simulink model "Aero_Dynamics"  (Simulink 8.3)
settings: Solver=ode45  StartTime=0.0  StopTime=10.0  RelTol=1e-3
values from neighbouring files (symbols this model uses):
  AD = [0.05526	0.05526	0.05568	0.05804	0.06460	0.08210 ... (first row only)    [AirCraftData.m]
  Alpha0 = [0.143	0.143	0.122	-0.267	-0.627	0.120 ... (first row only)    [AirCraftData.m]
  CA = 3.451    [AirCraftData.m]    (also in AircraftTrim.m)
  CDmin = [0.03799	0.03799	0.03799	0.03799	0.03904	0.04277 ... (first row only)    [AirCraftData.m]
  CLAlpha = [0.1012	0.1021	0.1033	0.1051	0.1079	0.0976 ... (first row only)    [AirCraftData.m]
  Clbt0 = [-0.00147	-0.00148	-0.00149	-0.00153	-0.00158	-0.00171 ... (first row only)    [AirCraftData.m]
  Clbtaf = [0	0	0	0	0	0;0	 0	0	0	0	0]    [AirCraftData.m]
  ClDelA = [-0.003110	-0.003065	-0.003040	-0.003036	-0.003052	-0.003088 ... (first row only)    [AirCraftData.m]
  CLDelE = [0.00653	0.00668	0.00690	0.00724	0.00772	0.00846 ... (first row only)    [AirCraftData.m]
  ClDelR = [0.000584	0.000605	0.000638	0.000686	0.000760	0.000877 ... (first row only)    [AirCraftData.m]
  CLDM = [0.244	0.244	0.244	0.244	0.244	0.244 ... (first row only)    [AirCraftData.m]
  Clp0 = [-0.5510 	-0.5610 	-0.5767 	-0.6005 	-0.6224 	-0.6763 ... (first row only)    [AirCraftData.m]
  ClpAf = [0,0,0,0,0,0;0,0,0,0,0,0]    [AirCraftData.m]
  Clr0 = [0.1308 	0.1339 	0.1383 	0.1474 	0.1601 	0.1738 ... (first row only)    [AirCraftData.m]
  ClrAf = [0,0,0,0,0,0;0,0,0,0,0,0]    [AirCraftData.m]
  Cm0 = [0.2014	0.2017	0.2034	0.2083	0.2207	0.2475 ... (first row only)    [AirCraftData.m]
  CmAfdot = [-11.5890 	-12.0169 	-12.7558 	-13.8010 	-15.2088 	-16.2278 ... (first row only)    [AirCraftData.m]
  CmCl = [-0.3454	-0.3441	-0.3427	-0.3412	-0.3396	-0.3379 ... (first row only)    [AirCraftData.m]
  CmDelE = [-0.03554	-0.03651	-0.03802	-0.04028	-0.04365	-0.04798 ... (first row only)    [AirCraftData.m]
  Cmq0 = [-42.0260 	-42.2665 	-42.9499 	-44.8315 	-45.5877 	-46.0842 ... (first row only)    [AirCraftData.m]
  CN1A0 = [0.0740	0.0662	0.0605	0.0552	0.0554 ... (first row only)    [AirCraftData.m]
  Cnbt0 = [0.00180	0.00183	0.00187	0.00192	0.00200	0.00207 ... (first row only)    [AirCraftData.m]
  Cnbtaf = [-0.000030 	-0.000031 	-0.000031 	-0.000032 	-0.000033 	-0.000035 ... (first row only)    [AirCraftData.m]
  CnDelA0 = [-0.000180	-0.000178	-0.000176	-0.000176	-0.000177	-0.000179 ... (first row only)    [AirCraftData.m]
  CnDelAAf = [0	 0	0	0	0	0;0	 0	0	0	0	0]    [AirCraftData.m]
  CnDelR = [-0.002214	-0.002274	-0.002367	-0.002505	-0.002712	-0.003039 ... (first row only)    [AirCraftData.m]
  Cnp0 = [0.0521 	0.0532 	0.0571 	0.0601 	0.0636 	0.0664 ... (first row only)    [AirCraftData.m]
  CnpAf = [0,0,0,0,0,0;0,0,0,0,0,0]    [AirCraftData.m]
  Cnr = [-0.1810 	-0.1832 	-0.1855 	-0.1892 	-0.1933 	-0.1973 ... (first row only)    [AirCraftData.m]
  Cxh_Slip = [0.0000, 0.0045, 0.0089, 0.0132, 0.0174 ... (first row only)    [AirCraftData.m]
  Cybeta0 = [-0.01783	-0.01790	-0.01804	-0.01824	-0.01851	-0.01884 ... (first row only)    [AirCraftData.m]
  Cybtaf = [0 0 0 0 0 0;0 0 0 0 0 0]    [AirCraftData.m]
  CyDelA = [0.000287	0.000295	0.000307	0.000325	0.000351	0.000394 ... (first row only)    [AirCraftData.m]
  CyDelR = [0.004946	0.005035	0.005316	0.005791	0.006458	0.007318 ... (first row only)    [AirCraftData.m]
  Cyh_Slip = [0.0000, -0.0248, -0.0519, -0.0813, -0.1130 ... (first row only)    [AirCraftData.m]
  ETA_data = [0.729 0.727 0.72 0.71 0.877 0.858 0.855 0.853 0.857 0.862 0.87 0.796 ... (330 elements, 11x5x6)]    [ETA_data.mat]
  eul_0 = [0/57.3 0/57.3 0/57.3]    [AircraftTrim.m]
  flap = 0    [AircraftTrim.m]
  inertia = [  Ix      Iy     Iz  Ixz]    [AircraftTrim.m]
  mass = 54000    [Start.m]    (also in drl_simplified_dynamics.m)
  Vab_0 = [Vt 0 0]    [AircraftTrim.m]
  Wxyz_0 = [0 0 0]    [AircraftTrim.m]
  X = 1.06    [AircraftTrim.m]
  xme_0 = [0 0 -alt]    [AircraftTrim.m]
  Y = 1.177    [AircraftTrim.m]
undefined symbols (not defined in the file or in its folder): slselsubs, thrust_data
libraries: aerolibatmos2 x1, aerolibobsolete x1, aerolibutil x1
(part 1 of 2)
settings Model: Creator=Administrator  LastModifiedBy=HP  BufferReuse=off
settings OptimizationCC: InlineParams=on  BufferReuse=off  ExpressionDepthLimit=2147483647  InitFltsAndDblsToZero=on
settings DebuggingCC: AlgebraicLoopMsg=none  SaveWithParameterizedLinksMsg=none  SignalResolutionControl=TryResolveAllWithWarning  SolverPrmCheckMsg=none  MultiTaskDSMMsg=warning  MultiTaskCondExecSysMsg=none  FcnCallInpInsideContextMsg=UseLocalSettings  UnconnectedInputMsg=none  UnconnectedOutputMsg=none  UnconnectedLineMsg=none  StrictBusMsg=Warning
settings RTWCC: IncludeERTFirstTime=on
settings GRTTargetCC: TargetFcnLib=ansi_tfl_tmw.mat

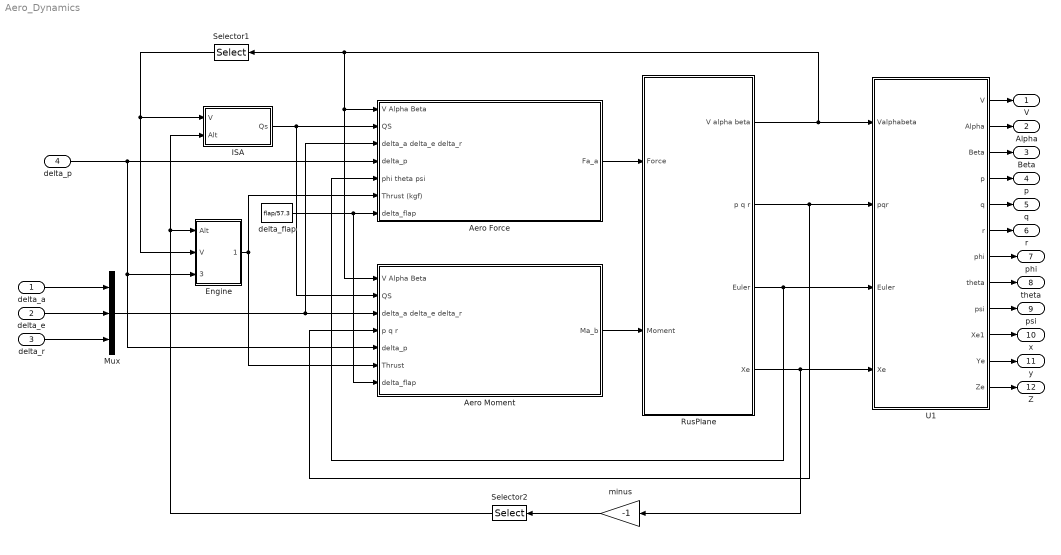
== system Aero_Dynamics ==
  delta_a : Inport
  delta_e : Inport  Port=2
  delta_r : Inport  Port=3
  delta_p : Inport  Port=4
  Aero Force : Subsystem
  Aero Moment : Subsystem
  Engine : Subsystem
  ISA : Subsystem
  Mux : Mux  Inputs=3
  RusPlane : Subsystem  mask{Xme_0=xme_0, Vab_0=Vab_0, eul_0=eul_0, Wxyz_0=Wxyz_0, inertia=inertia, mass=mass}
      mask prompts: Xme_0 "Initial position in inertial axes[Xe,Ye,Ze]"; Vab_0 "Initial velocity in body axes"; eul_0 "Initial Euler orientation"; Wxyz_0 "Initial body rotation rates"
  Selector1 : Selector  InputPortWidth=3  Indices=[1]  OutputSizes=[(-2)]
  Selector2 : Selector  InputPortWidth=3  Indices=[3]  OutputSizes=[(-2)]
  U1 : Subsystem
  delta_flap : Constant  Value=flap/57.3
  minus : Gain  Gain=-1
  V : Outport
  Alpha : Outport  Port=2
  Beta : Outport  Port=3
  p : Outport  Port=4
  q : Outport  Port=5
  r : Outport  Port=6
  phi : Outport  Port=7
  theta : Outport  Port=8
  psi : Outport  Port=9
  x : Outport  Port=10
  y : Outport  Port=11
  Z : Outport  Port=12
  wires:
  Aero Force/1(Fa_a) -> RusPlane/1(Force)
  Aero Moment/1(Ma_b) -> RusPlane/2(Moment)
  minus/1 -> Selector2/1
  RusPlane/1(V alpha beta) -> Aero Moment/1(V Alpha Beta), Aero Force/1(V Alpha Beta), Selector1/1, U1/1(Valphabeta)
  RusPlane/2(p q r) -> Aero Moment/4(p q r), U1/2(pqr)
  RusPlane/3(Euler) -> Aero Force/5(phi theta psi), U1/3(Euler)
  RusPlane/4(Xe) -> minus/1, U1/4(Xe)
  Selector1/1 -> ISA/1(V), Engine/2(V)
  ISA/1(Qs) -> Aero Force/2(QS), Aero Moment/2(QS)
  Engine/1(Thrust) -> Aero Force/6(Thrust (kgf)), Aero Moment/6(Thrust)
  Selector2/1 -> ISA/2(Alt), Engine/1(Alt)
  delta_a/1 -> Mux/1
  delta_e/1 -> Mux/2
  delta_r/1 -> Mux/3
  Mux/1 -> Aero Moment/3(delta_a delta_e delta_r), Aero Force/3(delta_a delta_e delta_r)
  delta_p/1 -> Aero Force/4(delta_p), Aero Moment/5(delta_p), Engine/3(delta_p)
  delta_flap/1 -> Aero Force/7(delta_flap), Aero Moment/7(delta_flap)
  U1/1(V) -> V/1
  U1/2(Alpha) -> Alpha/1
  U1/3(Beta) -> Beta/1
  U1/4(p) -> p/1
  U1/5(q) -> q/1
  U1/6(r) -> r/1
  U1/7(phi) -> phi/1
  U1/8(theta) -> theta/1
  U1/9(psi) -> psi/1
  U1/10(Xe1) -> x/1
  U1/11(Ye) -> y/1
  U1/12(Ze) -> Z/1

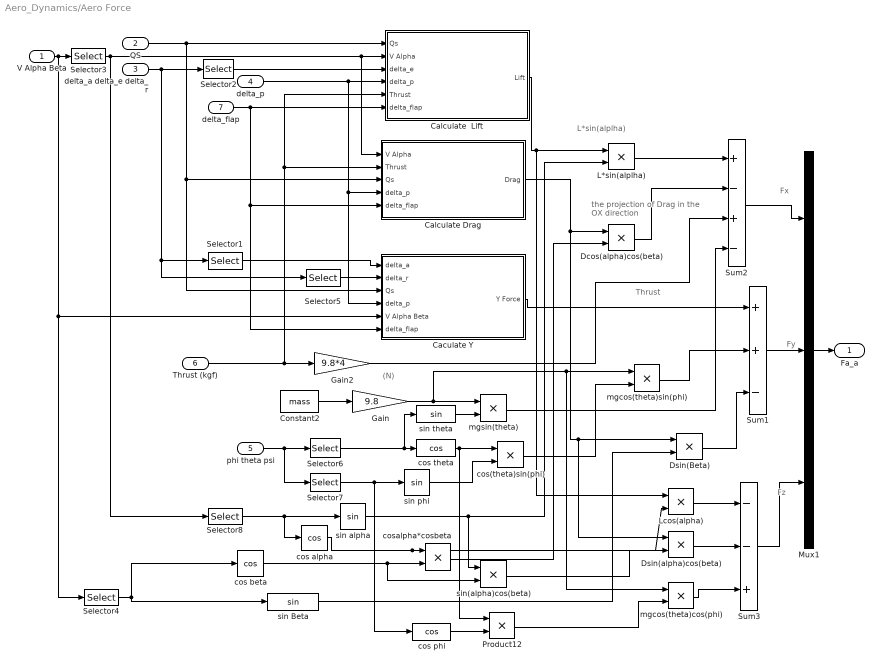
== system Aero_Dynamics/Aero Force ==
  note: Fx
  note: L*sin(alplha)
  note: the projection of Drag
      | in the OX direction
  note: Fy
  note: Fz
  note: Thrust
  note: (N)
  V Alpha Beta : Inport
  QS : Inport  Port=2
  delta_a delta_e delta_r : Inport  Port=3
  delta_p : Inport  Port=4
  phi theta psi : Inport  Port=5
  Thrust (kgf) : Inport  Port=6
  delta_flap : Inport  Port=7
  Caculate Y : Subsystem
  Calculate  Lift : Subsystem
  Calculate Drag : Subsystem
  Constant2 : Constant  Value=mass  OutDataTypeStr=Inherit: Inherit via back propagation
  Dcos(alpha)cos(beta) : Product  RndMeth=Zero
  Dsin(Beta) : Product  RndMeth=Zero
  Dsin(alpha)cos(beta) : Product  RndMeth=Zero
  Gain : Gain  Gain=9.8
  Gain2 : Gain  Gain=9.8*4
  L*sin(alplha) : Product  RndMeth=Zero
  Lcos(alpha) : Product  RndMeth=Zero
  Mux1 : Mux  Inputs=3
  Product12 : Product  RndMeth=Zero
  Selector1 : Selector  InputPortWidth=3  Indices=[1]  OutputSizes=[(-2)]
  Selector2 : Selector  InputPortWidth=3  Indices=[2]  OutputSizes=[(-2)]
  Selector3 : Selector  InputPortWidth=3  Indices=[1 2]  OutputSizes=[(-2)]
  Selector4 : Selector  InputPortWidth=3  Indices=[3]  OutputSizes=[(-2)]
  Selector5 : Selector  InputPortWidth=3  Indices=[3]  OutputSizes=[(-2)]
  Selector6 : Selector  InputPortWidth=3  Indices=[2]  OutputSizes=[(-2)]
  Selector7 : Selector  InputPortWidth=3  Indices=[1]  OutputSizes=[(-2)]
  Selector8 : Selector  InputPortWidth=2  Indices=[2]  OutputSizes=[(-2)]
  Sum1 : Sum  Inputs=++-
  Sum2 : Sum  Inputs=+-+-
  Sum3 : Sum  Inputs=--+
  cos alpha : Trigonometry  Operator=cos
  cos beta : Trigonometry  Operator=cos
  cos phi : Trigonometry  Operator=cos
  cos theta : Trigonometry  Operator=cos
  cos(theta)sin(phi) : Product  RndMeth=Zero
  cosalpha*cosbeta : Product  RndMeth=Zero
  mgcos(theta)cos(phi) : Product  RndMeth=Zero
  mgcos(theta)sin(phi) : Product  RndMeth=Zero
  mgsin(theta) : Product  RndMeth=Zero
  sin Beta : Trigonometry
  sin alpha : Trigonometry
  sin phi : Trigonometry
  sin theta : Trigonometry
  sin(alpha)cos(beta) : Product  RndMeth=Zero
  Fa_a : Outport
  wires:
  delta_a delta_e delta_r/1 -> Selector2/1, Selector5/1, Selector1/1
  Selector3/1 -> Selector8/1, Calculate  Lift/2(" V Alpha"), Calculate Drag/1(" V Alpha")
  Mux1/1 -> Fa_a/1
  Sum2/1 -> Mux1/1
  delta_p/1 -> Calculate Drag/4(delta_p), Caculate Y/4(delta_p), Calculate  Lift/4(delta_p)
  QS/1 -> Calculate  Lift/1(Qs), Calculate Drag/3(Qs), Caculate Y/3(Qs)
  Selector2/1 -> Calculate  Lift/3(delta_e)
  V Alpha Beta/1 -> Caculate Y/5(" V Alpha Beta"), Selector4/1, Selector3/1
  Calculate  Lift/1(Lift) -> L*sin(alplha)/1, Lcos(alpha)/1
  L*sin(alplha)/1 -> Sum2/1
  Calculate Drag/1(Drag) -> Dsin(Beta)/1, Dsin(alpha)cos(beta)/1, Dcos(alpha)cos(beta)/1
  cosalpha*cosbeta/1 -> Dcos(alpha)cos(beta)/2
  Dcos(alpha)cos(beta)/1 -> Sum2/2
  Thrust (kgf)/1 -> Gain2/1, Calculate  Lift/5(Thrust), Calculate Drag/2(Thrust)
  phi theta psi/1 -> Selector6/1, Selector7/1
  mgsin(theta)/1 -> Sum2/4
  Caculate Y/1(Y Force) -> Sum1/1
  Sum1/1 -> Mux1/2
  mgcos(theta)sin(phi)/1 -> Sum1/2
  Dsin(Beta)/1 -> Sum1/3
  Sum3/1 -> Mux1/3
  Lcos(alpha)/1 -> Sum3/1
  Dsin(alpha)cos(beta)/1 -> Sum3/2
  mgcos(theta)cos(phi)/1 -> Sum3/3
  Selector1/1 -> Caculate Y/1(delta_a)
  Selector5/1 -> Caculate Y/2(delta_r)
  Gain2/1 -> Sum2/3
  Selector8/1 -> sin alpha/1, cos alpha/1
  Product12/1 -> mgcos(theta)cos(phi)/2
  cos phi/1 -> Product12/2
  sin(alpha)cos(beta)/1 -> Dsin(alpha)cos(beta)/2
  sin Beta/1 -> Dsin(Beta)/2
  cos(theta)sin(phi)/1 -> mgcos(theta)sin(phi)/2
  cos theta/1 -> cos(theta)sin(phi)/1, Product12/1
  sin phi/1 -> cos(theta)sin(phi)/2
  Selector7/1 -> sin phi/1, cos phi/1
  cos beta/1 -> cosalpha*cosbeta/2, sin(alpha)cos(beta)/2
  cos alpha/1 -> cosalpha*cosbeta/1, Lcos(alpha)/2
  sin alpha/1 -> sin(alpha)cos(beta)/1, L*sin(alplha)/2
  sin theta/1 -> mgsin(theta)/2
  Selector6/1 -> sin theta/1, cos theta/1
  Gain/1 -> mgsin(theta)/1, mgcos(theta)sin(phi)/1, mgcos(theta)cos(phi)/1
  Constant2/1 -> Gain/1
  Selector4/1 -> cos beta/1, sin Beta/1
  delta_flap/1 -> Calculate  Lift/6(delta_flap), Calculate Drag/5(delta_flap), Caculate Y/6(delta_flap)

== system Aero_Dynamics/Aero Moment ==
  note: L
  note: M
  note: N
  V Alpha Beta : Inport
  QS : Inport  Port=2
  delta_a delta_e delta_r : Inport  Port=3
  p q r : Inport  Port=4
  delta_p : Inport  Port=5
  Thrust : Inport  Port=6
  delta_flap : Inport  Port=7
  Calculate Roll Moment L : Subsystem
  Calculate Yaw Moment N : Subsystem
  Calculate pitch Moment M : Subsystem
  Mux2 : Mux  Inputs=3
  Ma_b : Outport
  wires:
  Mux2/1 -> Ma_b/1
  QS/1 -> Calculate Roll Moment L/2(QS), Calculate pitch Moment M/1(QS), Calculate Yaw Moment N/2(QS)
  V Alpha Beta/1 -> Calculate Roll Moment L/1(V Alpha Beta), Calculate pitch Moment M/2(V alpha beta), Calculate Yaw Moment N/1(V Alpha Beta)
  delta_p/1 -> Calculate pitch Moment M/3(delta_p), Calculate Roll Moment L/5(delta_p), Calculate Yaw Moment N/5(delta_p)
  delta_a delta_e delta_r/1 -> Calculate Roll Moment L/3(delta_a delta_e delta_r), Calculate pitch Moment M/4(delta_a delta_e delta_r), Calculate Yaw Moment N/3(delta_a delta_e delta_r)
  p q r/1 -> Calculate Roll Moment L/4(p q r), Calculate pitch Moment M/5(p q r), Calculate Yaw Moment N/4(p q r)
  Calculate pitch Moment M/1(M) -> Mux2/2
  Calculate Roll Moment L/1(L) -> Mux2/1
  Calculate Yaw Moment N/1(N) -> Mux2/3
  Thrust/1 -> Calculate pitch Moment M/6(Thrust), Calculate Roll Moment L/6(Thrust)
  delta_flap/1 -> Calculate Roll Moment L/7(delta_flap), Calculate pitch Moment M/7(delta_flap), Calculate Yaw Moment N/6(delta_flap)

== system Aero_Dynamics/Engine ==
  Alt : Inport
  V : Inport  Port=2
  delta_p : Inport  Port=3
  Calculate Force : Lookup_n-D  NumberOfTableDimensions=3  BreakpointsForDimension1=[0,1000,2000,3000,4000,5000,6000,7000,8000,9000,10000]  BreakpointsForDimension2=[50,100,150,175,200]  BreakpointsForDimension3=[0.2,0.4,0.6,0.7,0.85,1,1.04]  BreakpointsForDimension5=slselsubs({[1:3], [1:3], [1:3], [1:3], [1:3], [1:3], [1:3], [1:3], [1:3], [1:3], [1:3], [1:3], [1:3], [1:3], [1:3], [1:3], [1:3], [1:3], [1:3], [1:3], [1:3], [1:3], [1:3], [1:3], [1:3], [1:3]}, 1)  BreakpointsForDimension6=slselsubs({[1:3], [1:3], [1:3], [1:3], [1:3], [1:3], [1:3], [1:3], [1:3], [1:3], [1:3], [1:3], [1:3], [1:3], [1:3], [1:3], [1:3], [1:3], [1:3], [1:3], [1:3], [1:3], [1:3], [1:3], [1:3], [1:3]}, 2)  BreakpointsForDimension7=slselsubs({[1:3], [1:3], [1:3], [1:3], [1:3], [1:3], [1:3], [1:3], [1:3], [1:3], [1:3], [1:3], [1:3], [1:3], [1:3], [1:3], [1:3], [1:3], [1:3], [1:3], [1:3], [1:3], [1:3], [1:3], [1:3], [1:3]}, 3)  BreakpointsForDimension8=slselsubs({[1:3], [1:3], [1:3], [1:3], [1:3], [1:3], [1:3], [1:3], [1:3], [1:3], [1:3], [1:3], [1:3], [1:3], [1:3], [1:3], [1:3], [1:3], [1:3], [1:3], [1:3], [1:3], [1:3], [1:3], [1:3], [1:3]}, 4)  BreakpointsForDimension9=slselsubs({[1:3], [1:3], [1:3], [1:3], [1:3], [1:3], [1:3], [1:3], [1:3], [1:3], [1:3], [1:3], [1:3], [1:3], [1:3], [1:3], [1:3], [1:3], [1:3], [1:3], [1:3], [1:3], [1:3], [1:3], [1:3], [1:3]}, 5)  BreakpointsForDimension10=slselsubs({[1:3], [1:3], [1:3], [1:3], [1:3], [1:3], [1:3], [1:3], [1:3], [1:3], [1:3], [1:3], [1:3], [1:3], [1:3], [1:3], [1:3], [1:3], [1:3], [1:3], [1:3], [1:3], [1:3], [1:3], [1:3], [1:3]}, 6)  BreakpointsForDimension11=slselsubs({[1:3], [1:3], [1:3], [1:3], [1:3], [1:3], [1:3], [1:3], [1:3], [1:3], [1:3], [1:3], [1:3], [1:3], [1:3], [1:3], [1:3], [1:3], [1:3], [1:3], [1:3], [1:3], [1:3], [1:3], [1:3], [1:3]}, 7)  BreakpointsForDimension12=slselsubs({[1:3], [1:3], [1:3], [1:3], [1:3], [1:3], [1:3], [1:3], [1:3], [1:3], [1:3], [1:3], [1:3], [1:3], [1:3], [1:3], [1:3], [1:3], [1:3], [1:3], [1:3], [1:3], [1:3], [1:3], [1:3], [1:3]}, 8)  BreakpointsForDimension13=slselsubs({[1:3], [1:3], [1:3], [1:3], [1:3], [1:3], [1:3], [1:3], [1:3], [1:3], [1:3], [1:3], [1:3], [1:3], [1:3], [1:3], [1:3], [1:3], [1:3], [1:3], [1:3], [1:3], [1:3], [1:3], [1:3], [1:3]}, 9)  BreakpointsForDimension14=slselsubs({[1:3], [1:3], [1:3], [1:3], [1:3], [1:3], [1:3], [1:3], [1:3], [1:3], [1:3], [1:3], [1:3], [1:3], [1:3], [1:3], [1:3], [1:3], [1:3], [1:3], [1:3], [1:3], [1:3], [1:3], [1:3], [1:3]}, 10)  BreakpointsForDimension15=slselsubs({[1:3], [1:3], [1:3], [1:3], [1:3], [1:3], [1:3], [1:3], [1:3], [1:3], [1:3], [1:3], [1:3], [1:3], [1:3], [1:3], [1:3], [1:3], [1:3], [1:3], [1:3], [1:3], [1:3], [1:3], [1:3], [1:3]}, 11)  BreakpointsForDimension16=slselsubs({[1:3], [1:3], [1:3], [1:3], [1:3], [1:3], [1:3], [1:3], [1:3], [1:3], [1:3], [1:3], [1:3], [1:3], [1:3], [1:3], [1:3], [1:3], [1:3], [1:3], [1:3], [1:3], [1:3], [1:3], [1:3], [1:3]}, 12)  BreakpointsForDimension17=slselsubs({[1:3], [1:3], [1:3], [1:3], [1:3], [1:3], [1:3], [1:3], [1:3], [1:3], [1:3], [1:3], [1:3], [1:3], [1:3], [1:3], [1:3], [1:3], [1:3], [1:3], [1:3], [1:3], [1:3], [1:3], [1:3], [1:3]}, 13)  BreakpointsForDimension18=slselsubs({[1:3], [1:3], [1:3], [1:3], [1:3], [1:3], [1:3], [1:3], [1:3], [1:3], [1:3], [1:3], [1:3], [1:3], [1:3], [1:3], [1:3], [1:3], [1:3], [1:3], [1:3], [1:3], [1:3], [1:3], [1:3], [1:3]}, 14)  BreakpointsForDimension19=slselsubs({[1:3], [1:3], [1:3], [1:3], [1:3], [1:3], [1:3], [1:3], [1:3], [1:3], [1:3], [1:3], [1:3], [1:3], [1:3], [1:3], [1:3], [1:3], [1:3], [1:3], [1:3], [1:3], [1:3], [1:3], [1:3], [1:3]}, 15)  BreakpointsForDimension20=slselsubs({[1:3], [1:3], [1:3], [1:3], [1:3], [1:3], [1:3], [1:3], [1:3], [1:3], [1:3], [1:3], [1:3], [1:3], [1:3], [1:3], [1:3], [1:3], [1:3], [1:3], [1:3], [1:3], [1:3], [1:3], [1:3], [1:3]}, 16)  BreakpointsForDimension21=slselsubs({[1:3], [1:3], [1:3], [1:3], [1:3], [1:3], [1:3], [1:3], [1:3], [1:3], [1:3], [1:3], [1:3], [1:3], [1:3], [1:3], [1:3], [1:3], [1:3], [1:3], [1:3], [1:3], [1:3], [1:3], [1:3], [1:3]}, 17)  BreakpointsForDimension22=slselsubs({[1:3], [1:3], [1:3], [1:3], [1:3], [1:3], [1:3], [1:3], [1:3], [1:3], [1:3], [1:3], [1:3], [1:3], [1:3], [1:3], [1:3], [1:3], [1:3], [1:3], [1:3], [1:3], [1:3], [1:3], [1:3], [1:3]}, 18)  BreakpointsForDimension23=slselsubs({[1:3], [1:3], [1:3], [1:3], [1:3], [1:3], [1:3], [1:3], [1:3], [1:3], [1:3], [1:3], [1:3], [1:3], [1:3], [1:3], [1:3], [1:3], [1:3], [1:3], [1:3], [1:3], [1:3], [1:3], [1:3], [1:3]}, 19)  BreakpointsForDimension24=slselsubs({[1:3], [1:3], [1:3], [1:3], [1:3], [1:3], [1:3], [1:3], [1:3], [1:3], [1:3], [1:3], [1:3], [1:3], [1:3], [1:3], [1:3], [1:3], [1:3], [1:3], [1:3], [1:3], [1:3], [1:3], [1:3], [1:3]}, 20)  BreakpointsForDimension25=slselsubs({[1:3], [1:3], [1:3], [1:3], [1:3], [1:3], [1:3], [1:3], [1:3], [1:3], [1:3], [1:3], [1:3], [1:3], [1:3], [1:3], [1:3], [1:3], [1:3], [1:3], [1:3], [1:3], [1:3], [1:3], [1:3], [1:3]}, 21)  BreakpointsForDimension26=slselsubs({[1:3], [1:3], [1:3], [1:3], [1:3], [1:3], [1:3], [1:3], [1:3], [1:3], [1:3], [1:3], [1:3], [1:3], [1:3], [1:3], [1:3], [1:3], [1:3], [1:3], [1:3], [1:3], [1:3], [1:3], [1:3], [1:3]}, 22)  BreakpointsForDimension27=slselsubs({[1:3], [1:3], [1:3], [1:3], [1:3], [1:3], [1:3], [1:3], [1:3], [1:3], [1:3], [1:3], [1:3], [1:3], [1:3], [1:3], [1:3], [1:3], [1:3], [1:3], [1:3], [1:3], [1:3], [1:3], [1:3], [1:3]}, 23)  BreakpointsForDimension28=slselsubs({[1:3], [1:3], [1:3], [1:3], [1:3], [1:3], [1:3], [1:3], [1:3], [1:3], [1:3], [1:3], [1:3], [1:3], [1:3], [1:3], [1:3], [1:3], [1:3], [1:3], [1:3], [1:3], [1:3], [1:3], [1:3], [1:3]}, 24)  BreakpointsForDimension29=slselsubs({[1:3], [1:3], [1:3], [1:3], [1:3], [1:3], [1:3], [1:3], [1:3], [1:3], [1:3], [1:3], [1:3], [1:3], [1:3], [1:3], [1:3], [1:3], [1:3], [1:3], [1:3], [1:3], [1:3], [1:3], [1:3], [1:3]}, 25)  BreakpointsForDimension30=slselsubs({[1:3], [1:3], [1:3], [1:3], [1:3], [1:3], [1:3], [1:3], [1:3], [1:3], [1:3], [1:3], [1:3], [1:3], [1:3], [1:3], [1:3], [1:3], [1:3], [1:3], [1:3], [1:3], [1:3], [1:3], [1:3], [1:3]}, 26)  Table=thrust_data  InterpMethod=Cubic spline  ExtrapMethod=Cubic spline  InputSameDT=on
  Thrust : Outport
  wires:
  Calculate Force/1 -> Thrust/1
  delta_p/1 -> Calculate Force/3
  Alt/1 -> Calculate Force/1
  V/1 -> Calculate Force/2

== system Aero_Dynamics/ISA ==
  note: V
  note: V^2
  V : Inport
  Alt : Inport  Port=2
  Constant2 : Constant  Value=0.5
  Divide : Product  Inputs=/*
  ISA Atmosphere Model : aerolibatmos2/ISA Atmosphere Model  SystemSampleTime=-1  custom=off  g=9.80665  gamma=1.4  R=287.0531  L=0.0065  h_trop=11000  h_strat=20000  rho0=1.225  P0=101325  T0=288.15
  Product : Product  Inputs=3  RndMeth=Zero
  Product2 : Product  RndMeth=Zero
  Scope1 : Scope
  Scope2 : Scope
      settings: SaveName=ScopeData2
  To Workspace : ToWorkspace  VariableName=Rou  SampleTime=-1
  Qs : Outport
  tag scope: Alt=global, Ma=global
  wires:
  ISA Atmosphere Model/4 -> To Workspace/1, Product/1
  Alt/1 -> ISA Atmosphere Model/1, [Alt]
  ISA Atmosphere Model/1 -> Scope2/1
  ISA Atmosphere Model/3 -> Scope1/1
  Product/1 -> Qs/1
  Divide/1 -> [Ma]
  ISA Atmosphere Model/2 -> Divide/1
  Product2/1 -> Product/3
  Constant2/1 -> Product/2
  V/1 -> Divide/2, Product2/1, Product2/2

== system Aero_Dynamics/RusPlane ==
  Force : Inport
  Moment : Inport  Port=2
  AV Alpha Beta : Subsystem
  BWxyz2 : Integrator  InitialCondition=Wxyz_0
  Calculate DCM & Euler Angles : Subsystem  AncestorBlock=aerolib6dofsys/DCM & Euler Angles (Euler)  mask(DCM & Euler Angles (Euler)){}
  Constant1 : Constant  Value=inertia  OutDataTypeStr=Inherit: Inherit via back propagation
  Constant2 : Constant  Value=mass  OutDataTypeStr=Inherit: Inherit via back propagation
  Product : Product  Inputs=*/  SaturateOnIntegerOverflow=on  OutDataTypeStr=Inherit: Same as first input
  Subsystem : Subsystem
  Subsystem1 : Subsystem
  Sum : Sum  Inputs=|++  SaturateOnIntegerOverflow=on
  Vbxw : aerolibutil/3x3 Cross Product
  xe,ye,ze : Integrator  InitialCondition=xme_0
  V alpha beta : Outport
  p q r : Outport  Port=2
  Euler : Outport  Port=3
  Xe : Outport  Port=4
  wires:
  Constant1/1 -> Subsystem/3(inertia Ix Iy Iz Ixz)
  Product/1 -> Sum/1
  Sum/1 -> AV Alpha Beta/1(udot vdot wdot)
  Vbxw/1 -> Sum/2
  Constant2/1 -> Product/2
  BWxyz2/1 -> Calculate DCM & Euler Angles/1("Wxyz "), p q r/1, Vbxw/2, Subsystem/2(pqr)  "pqr"
  Subsystem1/1(Xedot Yedot Zedot) -> xe,ye,ze/1
  Force/1 -> Product/1  "Force"
  xe,ye,ze/1 -> Xe/1  "Xe"
  Calculate DCM & Euler Angles/1(Euler) -> Euler/1, Subsystem1/2(Euler phi  theta  psi)  "Eular"
  AV Alpha Beta/2(u v w  in) -> Vbxw/1, Subsystem1/1("U V W ")
  AV Alpha Beta/1(V alpha beta) -> V alpha beta/1
  Subsystem/1(pdot qdot rdot) -> BWxyz2/1
  Moment/1 -> Subsystem/1(Moment L M N)  "Moment"

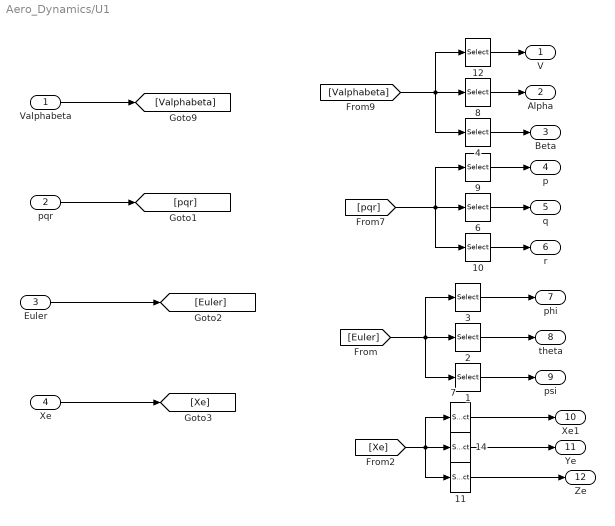
== system Aero_Dynamics/U1 ==
  Valphabeta : Inport
  pqr : Inport  Port=2
  Euler : Inport  Port=3
  Xe : Inport  Port=4
  {1,4,10..11} (4 alike) : Selector  InputPortWidth=3  Indices=3  OutputSizes=[(-2)]
  {3,7,9,12} (4 alike) : Selector  InputPortWidth=3  OutputSizes=[(-2)]
  {2,6,8,14} (4 alike) : Selector  InputPortWidth=3  Indices=2  OutputSizes=[(-2)]
  V : Outport
  Alpha : Outport  Port=2
  Beta : Outport  Port=3
  p : Outport  Port=4
  q : Outport  Port=5
  r : Outport  Port=6
  phi : Outport  Port=7
  theta : Outport  Port=8
  psi : Outport  Port=9
  Xe1 : Outport  Port=10
  Ye : Outport  Port=11
  Ze : Outport  Port=12
  wires:
  7/1 -> Xe1/1
  [Xe] -> 11/1, 14/1, 7/1
  11/1 -> Ze/1
  14/1 -> Ye/1
  10/1 -> r/1
  [pqr] -> 6/1, 9/1, 10/1
  9/1 -> p/1
  6/1 -> q/1
  1/1 -> psi/1
  [Euler] -> 2/1, 3/1, 1/1
  3/1 -> phi/1
  2/1 -> theta/1
  4/1 -> Beta/1
  [Valphabeta] -> 8/1, 12/1, 4/1
  12/1 -> V/1
  8/1 -> Alpha/1
  Valphabeta/1 -> [Valphabeta]
  pqr/1 -> [pqr]
  Euler/1 -> [Euler]
  Xe/1 -> [Xe]

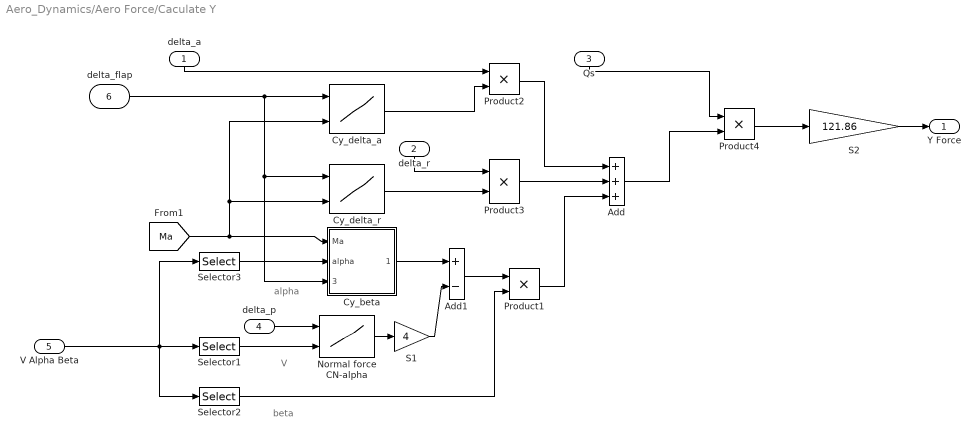
== system Aero_Dynamics/Aero Force/Caculate Y ==
  note: V
  note: beta
  note: alpha
  delta_a : Inport
  delta_r : Inport  Port=2
  Qs : Inport  Port=3
  delta_p : Inport  Port=4
  " V Alpha Beta" : Inport  Port=5
  delta_flap : Inport  Port=6
  Add : Sum  Inputs=+++
  Add1 : Sum  Inputs=+-
  Cy_beta : Subsystem
  Cy_delta_a : Lookup2D  RowIndex=[0 6/57.3]  ColumnIndex=Mach_table  Table=CyDelA
  Cy_delta_r : Lookup2D  RowIndex=[0 6/57.3]  ColumnIndex=Mach_table  Table=CyDelR
  Normal force CN-alpha : Lookup2D  RowIndex=[0.4,0.7,0.85,1,1.04]  ColumnIndex=[50,75,100,150,175]  Table=CN1A0
  Product{1..4} (4 alike) : Product  RndMeth=Zero
  S1 : Gain  Gain=4
  S2 : Gain  Gain=121.86
  Selector1 : Selector  InputPortWidth=3  Indices=[1]  OutputSizes=[(-2)]
  Selector2 : Selector  InputPortWidth=3  Indices=[3]  OutputSizes=[(-2)]
  Selector3 : Selector  InputPortWidth=3  Indices=[2]  OutputSizes=[(-2)]
  Y Force : Outport
  wires:
  [Ma] -> Cy_delta_a/2, Cy_delta_r/2, Cy_beta/1(Ma)
  Cy_delta_a/1 -> Product2/2
  Cy_delta_r/1 -> Product3/2
  Product2/1 -> Add/1
  Product3/1 -> Add/2
  Product1/1 -> Add/3
  Add/1 -> Product4/2
  delta_a/1 -> Product2/1
  Qs/1 -> Product4/1
  Product4/1 -> S2/1
  Selector2/1 -> Product1/2
  delta_r/1 -> Product3/1
  " V Alpha Beta"/1 -> Selector1/1, Selector2/1, Selector3/1
  Selector3/1 -> Cy_beta/2(alpha)
  Cy_beta/1(Cybeta) -> Add1/1
  Add1/1 -> Product1/1
  Normal force CN-alpha/1 -> S1/1
  delta_p/1 -> Normal force CN-alpha/1
  Selector1/1 -> Normal force CN-alpha/2
  S2/1 -> Y Force/1
  S1/1 -> Add1/2
  delta_flap/1 -> Cy_delta_a/1, Cy_delta_r/1, Cy_beta/3(delta_flap)

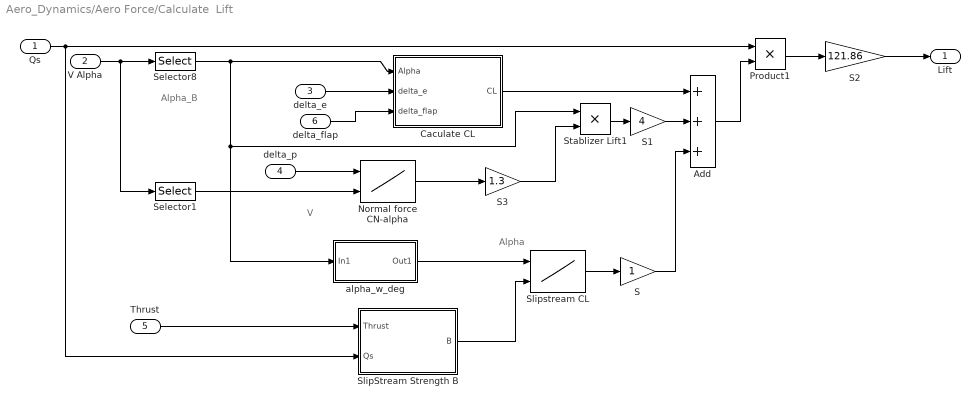
== system Aero_Dynamics/Aero Force/Calculate  Lift ==
  note: Alpha
  note: Alpha_B
  note: V
  Qs : Inport
  " V Alpha" : Inport  Port=2
  delta_e : Inport  Port=3
  delta_p : Inport  Port=4
  Thrust : Inport  Port=5
  delta_flap : Inport  Port=6
  Add : Sum  Inputs=+++
  Caculate CL : Subsystem
  Normal force CN-alpha : Lookup2D  RowIndex=[0.4,0.7,0.85,1,1.04]  ColumnIndex=[50,75,100,150,175]  Table=CN1A0
  Product1 : Product  RndMeth=Zero
  S : Gain
  S1 : Gain  Gain=4
  S2 : Gain  Gain=121.86
  S3 : Gain  Gain=1.3
  Selector1 : Selector  InputPortWidth=2  Indices=[1]  OutputSizes=[(-2)]
  Selector8 : Selector  InputPortWidth=2  Indices=[2]  OutputSizes=[(-2)]
  SlipStream Strength B : Subsystem
  Slipstream CL : Lookup2D  RowIndex=[0,2,4,6,8,10,12,14,16 18]  ColumnIndex=[0 0.25 0.5 0.75 1]  Table=Cyh_Slip
  Stablizer Lift1 : Product  RndMeth=Zero
  alpha_w_deg : Subsystem
  Lift : Outport
  wires:
  Add/1 -> Product1/2
  Selector1/1 -> Normal force CN-alpha/2
  Stablizer Lift1/1 -> S1/1
  " V Alpha"/1 -> Selector8/1, Selector1/1
  Qs/1 -> Product1/1, SlipStream Strength B/2(Qs)
  Product1/1 -> S2/1
  SlipStream Strength B/1(B) -> Slipstream CL/2
  Slipstream CL/1 -> S/1
  S/1 -> Add/3
  S1/1 -> Add/2
  Selector8/1 -> Caculate CL/1(Alpha), Stablizer Lift1/1, alpha_w_deg/1(In1)
  Thrust/1 -> SlipStream Strength B/1(Thrust)
  delta_e/1 -> Caculate CL/2(delta_e)
  Caculate CL/1(CL) -> Add/1
  Normal force CN-alpha/1 -> S3/1
  delta_p/1 -> Normal force CN-alpha/1
  S2/1 -> Lift/1
  alpha_w_deg/1(Out1) -> Slipstream CL/1
  S3/1 -> Stablizer Lift1/2
  delta_flap/1 -> Caculate CL/3(delta_flap)

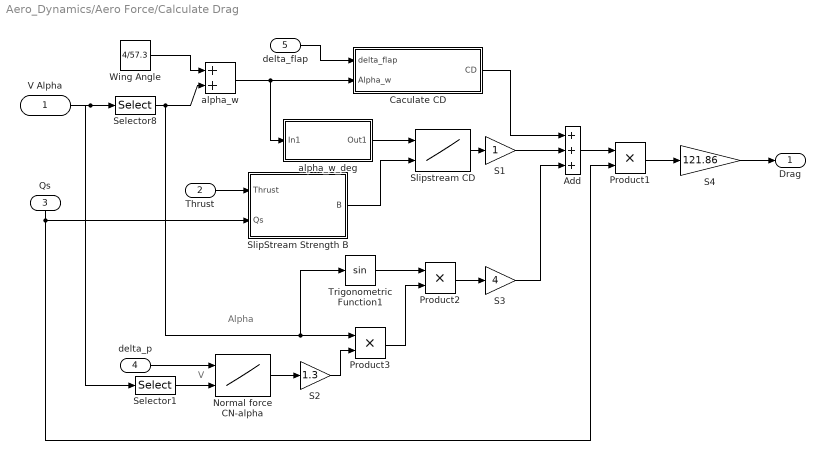
== system Aero_Dynamics/Aero Force/Calculate Drag ==
  note: V
  note: Alpha
  " V Alpha" : Inport
  Thrust : Inport  Port=2
  Qs : Inport  Port=3
  delta_p : Inport  Port=4
  delta_flap : Inport  Port=5
  Add : Sum  Inputs=+++
  "Caculate CD " : Subsystem
  Normal force CN-alpha : Lookup2D  RowIndex=[0.4,0.7,0.85,1,1.04]  ColumnIndex=[50,75,100,150,175]  Table=CN1A0
  Product1 : Product  RndMeth=Zero
  Product2 : Product  RndMeth=Zero
  Product3 : Product  RndMeth=Zero
  S1 : Gain
  S2 : Gain  Gain=1.3
  S3 : Gain  Gain=4
  S4 : Gain  Gain=121.86
  Selector1 : Selector  InputPortWidth=2  Indices=[1]  OutputSizes=[(-2)]
  Selector8 : Selector  InputPortWidth=2  Indices=[2]  OutputSizes=[(-2)]
  SlipStream Strength B : Subsystem
  Slipstream CD : Lookup2D  RowIndex=[0,2,4,6,8,10,12,14,16,18]  ColumnIndex=[0,0.25,0.5,0.75,1]  Table=Cxh_Slip
  Trigonometric Function1 : Trigonometry
  Wing Angle : Constant  Value=4/57.3
  alpha_w : Sum
  alpha_w_deg : Subsystem
  Drag : Outport
  wires:
  SlipStream Strength B/1(B) -> Slipstream CD/2
  Slipstream CD/1 -> S1/1
  Add/1 -> Product1/1
  S1/1 -> Add/2
  " V Alpha"/1 -> Selector8/1, Selector1/1
  Thrust/1 -> SlipStream Strength B/1(Thrust)
  Qs/1 -> SlipStream Strength B/2(Qs), Product1/2
  Product1/1 -> S4/1
  "Caculate CD "/1(CD) -> Add/1
  alpha_w_deg/1(Out1) -> Slipstream CD/1
  alpha_w/1 -> "Caculate CD "/2("  Alpha_w"), alpha_w_deg/1(In1)
  Wing Angle/1 -> alpha_w/1
  Selector8/1 -> alpha_w/2, Product3/1, Trigonometric Function1/1
  Normal force CN-alpha/1 -> S2/1
  Product3/1 -> Product2/2
  Trigonometric Function1/1 -> Product2/1
  Product2/1 -> S3/1
  S3/1 -> Add/3
  delta_p/1 -> Normal force CN-alpha/1
  Selector1/1 -> Normal force CN-alpha/2
  S4/1 -> Drag/1
  S2/1 -> Product3/2
  delta_flap/1 -> "Caculate CD "/1(" delta_flap")

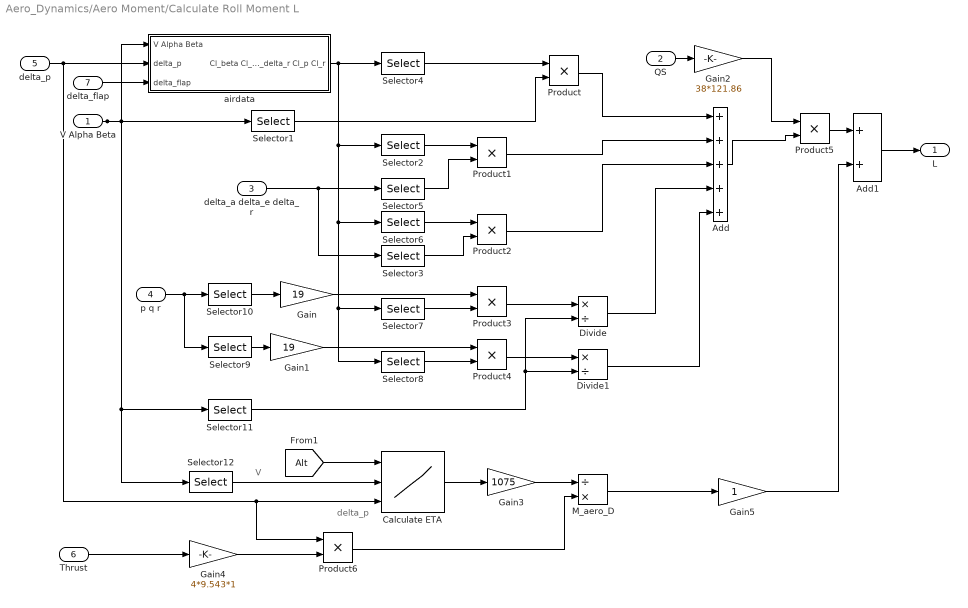
== system Aero_Dynamics/Aero Moment/Calculate Roll Moment L ==
  note: V
  note: delta_p
  V Alpha Beta : Inport
  QS : Inport  Port=2
  delta_a delta_e delta_r : Inport  Port=3
  p q r : Inport  Port=4
  delta_p : Inport  Port=5
  Thrust : Inport  Port=6
  delta_flap : Inport  Port=7
  Add : Sum  Inputs=+++++
  Add1 : Sum
  Calculate ETA : Lookup_n-D  NumberOfTableDimensions=3  BreakpointsForDimension1=[0,1000,2000,3000,4000,5000,6000,7000,8000,9000,10000]  BreakpointsForDimension2=[50,100,150,175,200]  BreakpointsForDimension3=[0.4,0.6,0.7,0.85,1,1.04]  BreakpointsForDimension5=slselsubs({[1:3], [1:3], [1:3], [1:3], [1:3], [1:3], [1:3], [1:3], [1:3], [1:3], [1:3], [1:3], [1:3], [1:3], [1:3], [1:3], [1:3], [1:3], [1:3], [1:3], [1:3], [1:3], [1:3], [1:3], [1:3], [1:3]}, 1)  BreakpointsForDimension6=slselsubs({[1:3], [1:3], [1:3], [1:3], [1:3], [1:3], [1:3], [1:3], [1:3], [1:3], [1:3], [1:3], [1:3], [1:3], [1:3], [1:3], [1:3], [1:3], [1:3], [1:3], [1:3], [1:3], [1:3], [1:3], [1:3], [1:3]}, 2)  BreakpointsForDimension7=slselsubs({[1:3], [1:3], [1:3], [1:3], [1:3], [1:3], [1:3], [1:3], [1:3], [1:3], [1:3], [1:3], [1:3], [1:3], [1:3], [1:3], [1:3], [1:3], [1:3], [1:3], [1:3], [1:3], [1:3], [1:3], [1:3], [1:3]}, 3)  BreakpointsForDimension8=slselsubs({[1:3], [1:3], [1:3], [1:3], [1:3], [1:3], [1:3], [1:3], [1:3], [1:3], [1:3], [1:3], [1:3], [1:3], [1:3], [1:3], [1:3], [1:3], [1:3], [1:3], [1:3], [1:3], [1:3], [1:3], [1:3], [1:3]}, 4)  BreakpointsForDimension9=slselsubs({[1:3], [1:3], [1:3], [1:3], [1:3], [1:3], [1:3], [1:3], [1:3], [1:3], [1:3], [1:3], [1:3], [1:3], [1:3], [1:3], [1:3], [1:3], [1:3], [1:3], [1:3], [1:3], [1:3], [1:3], [1:3], [1:3]}, 5)  BreakpointsForDimension10=slselsubs({[1:3], [1:3], [1:3], [1:3], [1:3], [1:3], [1:3], [1:3], [1:3], [1:3], [1:3], [1:3], [1:3], [1:3], [1:3], [1:3], [1:3], [1:3], [1:3], [1:3], [1:3], [1:3], [1:3], [1:3], [1:3], [1:3]}, 6)  BreakpointsForDimension11=slselsubs({[1:3], [1:3], [1:3], [1:3], [1:3], [1:3], [1:3], [1:3], [1:3], [1:3], [1:3], [1:3], [1:3], [1:3], [1:3], [1:3], [1:3], [1:3], [1:3], [1:3], [1:3], [1:3], [1:3], [1:3], [1:3], [1:3]}, 7)  BreakpointsForDimension12=slselsubs({[1:3], [1:3], [1:3], [1:3], [1:3], [1:3], [1:3], [1:3], [1:3], [1:3], [1:3], [1:3], [1:3], [1:3], [1:3], [1:3], [1:3], [1:3], [1:3], [1:3], [1:3], [1:3], [1:3], [1:3], [1:3], [1:3]}, 8)  BreakpointsForDimension13=slselsubs({[1:3], [1:3], [1:3], [1:3], [1:3], [1:3], [1:3], [1:3], [1:3], [1:3], [1:3], [1:3], [1:3], [1:3], [1:3], [1:3], [1:3], [1:3], [1:3], [1:3], [1:3], [1:3], [1:3], [1:3], [1:3], [1:3]}, 9)  BreakpointsForDimension14=slselsubs({[1:3], [1:3], [1:3], [1:3], [1:3], [1:3], [1:3], [1:3], [1:3], [1:3], [1:3], [1:3], [1:3], [1:3], [1:3], [1:3], [1:3], [1:3], [1:3], [1:3], [1:3], [1:3], [1:3], [1:3], [1:3], [1:3]}, 10)  BreakpointsForDimension15=slselsubs({[1:3], [1:3], [1:3], [1:3], [1:3], [1:3], [1:3], [1:3], [1:3], [1:3], [1:3], [1:3], [1:3], [1:3], [1:3], [1:3], [1:3], [1:3], [1:3], [1:3], [1:3], [1:3], [1:3], [1:3], [1:3], [1:3]}, 11)  BreakpointsForDimension16=slselsubs({[1:3], [1:3], [1:3], [1:3], [1:3], [1:3], [1:3], [1:3], [1:3], [1:3], [1:3], [1:3], [1:3], [1:3], [1:3], [1:3], [1:3], [1:3], [1:3], [1:3], [1:3], [1:3], [1:3], [1:3], [1:3], [1:3]}, 12)  BreakpointsForDimension17=slselsubs({[1:3], [1:3], [1:3], [1:3], [1:3], [1:3], [1:3], [1:3], [1:3], [1:3], [1:3], [1:3], [1:3], [1:3], [1:3], [1:3], [1:3], [1:3], [1:3], [1:3], [1:3], [1:3], [1:3], [1:3], [1:3], [1:3]}, 13)  BreakpointsForDimension18=slselsubs({[1:3], [1:3], [1:3], [1:3], [1:3], [1:3], [1:3], [1:3], [1:3], [1:3], [1:3], [1:3], [1:3], [1:3], [1:3], [1:3], [1:3], [1:3], [1:3], [1:3], [1:3], [1:3], [1:3], [1:3], [1:3], [1:3]}, 14)  BreakpointsForDimension19=slselsubs({[1:3], [1:3], [1:3], [1:3], [1:3], [1:3], [1:3], [1:3], [1:3], [1:3], [1:3], [1:3], [1:3], [1:3], [1:3], [1:3], [1:3], [1:3], [1:3], [1:3], [1:3], [1:3], [1:3], [1:3], [1:3], [1:3]}, 15)  BreakpointsForDimension20=slselsubs({[1:3], [1:3], [1:3], [1:3], [1:3], [1:3], [1:3], [1:3], [1:3], [1:3], [1:3], [1:3], [1:3], [1:3], [1:3], [1:3], [1:3], [1:3], [1:3], [1:3], [1:3], [1:3], [1:3], [1:3], [1:3], [1:3]}, 16)  BreakpointsForDimension21=slselsubs({[1:3], [1:3], [1:3], [1:3], [1:3], [1:3], [1:3], [1:3], [1:3], [1:3], [1:3], [1:3], [1:3], [1:3], [1:3], [1:3], [1:3], [1:3], [1:3], [1:3], [1:3], [1:3], [1:3], [1:3], [1:3], [1:3]}, 17)  BreakpointsForDimension22=slselsubs({[1:3], [1:3], [1:3], [1:3], [1:3], [1:3], [1:3], [1:3], [1:3], [1:3], [1:3], [1:3], [1:3], [1:3], [1:3], [1:3], [1:3], [1:3], [1:3], [1:3], [1:3], [1:3], [1:3], [1:3], [1:3], [1:3]}, 18)  BreakpointsForDimension23=slselsubs({[1:3], [1:3], [1:3], [1:3], [1:3], [1:3], [1:3], [1:3], [1:3], [1:3], [1:3], [1:3], [1:3], [1:3], [1:3], [1:3], [1:3], [1:3], [1:3], [1:3], [1:3], [1:3], [1:3], [1:3], [1:3], [1:3]}, 19)  BreakpointsForDimension24=slselsubs({[1:3], [1:3], [1:3], [1:3], [1:3], [1:3], [1:3], [1:3], [1:3], [1:3], [1:3], [1:3], [1:3], [1:3], [1:3], [1:3], [1:3], [1:3], [1:3], [1:3], [1:3], [1:3], [1:3], [1:3], [1:3], [1:3]}, 20)  BreakpointsForDimension25=slselsubs({[1:3], [1:3], [1:3], [1:3], [1:3], [1:3], [1:3], [1:3], [1:3], [1:3], [1:3], [1:3], [1:3], [1:3], [1:3], [1:3], [1:3], [1:3], [1:3], [1:3], [1:3], [1:3], [1:3], [1:3], [1:3], [1:3]}, 21)  BreakpointsForDimension26=slselsubs({[1:3], [1:3], [1:3], [1:3], [1:3], [1:3], [1:3], [1:3], [1:3], [1:3], [1:3], [1:3], [1:3], [1:3], [1:3], [1:3], [1:3], [1:3], [1:3], [1:3], [1:3], [1:3], [1:3], [1:3], [1:3], [1:3]}, 22)  BreakpointsForDimension27=slselsubs({[1:3], [1:3], [1:3], [1:3], [1:3], [1:3], [1:3], [1:3], [1:3], [1:3], [1:3], [1:3], [1:3], [1:3], [1:3], [1:3], [1:3], [1:3], [1:3], [1:3], [1:3], [1:3], [1:3], [1:3], [1:3], [1:3]}, 23)  BreakpointsForDimension28=slselsubs({[1:3], [1:3], [1:3], [1:3], [1:3], [1:3], [1:3], [1:3], [1:3], [1:3], [1:3], [1:3], [1:3], [1:3], [1:3], [1:3], [1:3], [1:3], [1:3], [1:3], [1:3], [1:3], [1:3], [1:3], [1:3], [1:3]}, 24)  BreakpointsForDimension29=slselsubs({[1:3], [1:3], [1:3], [1:3], [1:3], [1:3], [1:3], [1:3], [1:3], [1:3], [1:3], [1:3], [1:3], [1:3], [1:3], [1:3], [1:3], [1:3], [1:3], [1:3], [1:3], [1:3], [1:3], [1:3], [1:3], [1:3]}, 25)  BreakpointsForDimension30=slselsubs({[1:3], [1:3], [1:3], [1:3], [1:3], [1:3], [1:3], [1:3], [1:3], [1:3], [1:3], [1:3], [1:3], [1:3], [1:3], [1:3], [1:3], [1:3], [1:3], [1:3], [1:3], [1:3], [1:3], [1:3], [1:3], [1:3]}, 26)  Table=ETA_data  InterpMethod=Cubic spline  ExtrapMethod=Cubic spline  InputSameDT=on
  Divide : Product  Inputs=*/
  Divide1 : Product  Inputs=*/
  Gain : Gain  Gain=19
  Gain1 : Gain  Gain=19
  Gain2 : Gain  Gain=38*121.86
  Gain3 : Gain  Gain=1075
  Gain4 : Gain  Gain=4*9.543*1
  Gain5 : Gain
  M_aero_D : Product  Inputs=/*
  Product{,1..6} (7 alike) : Product  RndMeth=Zero
  Selector1 : Selector  InputPortWidth=3  Indices=[3]  OutputSizes=[(-2)]
  Selector{5,10..12} (4 alike) : Selector  InputPortWidth=3  Indices=[1]  OutputSizes=[(-2)]
  Selector2 : Selector  InputPortWidth=5  Indices=[2]  OutputSizes=[(-2)]
  Selector3 : Selector  InputPortWidth=3  Indices=[3]  OutputSizes=[(-2)]
  Selector4 : Selector  InputPortWidth=5  Indices=[1]  OutputSizes=[(-2)]
  Selector6 : Selector  InputPortWidth=5  Indices=[3]  OutputSizes=[(-2)]
  Selector7 : Selector  InputPortWidth=5  Indices=[4]  OutputSizes=[(-2)]
  Selector8 : Selector  InputPortWidth=5  Indices=[5]  OutputSizes=[(-2)]
  Selector9 : Selector  InputPortWidth=3  Indices=[3]  OutputSizes=[(-2)]
  airdata : Subsystem
  L : Outport
  wires:
  airdata/1(Cl_beta Cl_delta_a Cl_delta_r Cl_p Cl_r) -> Selector4/1, Selector2/1, Selector6/1, Selector7/1, Selector8/1
  V Alpha Beta/1 -> Selector1/1, Selector11/1, Selector12/1, airdata/1(V Alpha Beta)
  Selector4/1 -> Product/1
  Selector1/1 -> Product/2
  Selector2/1 -> Product1/1
  delta_a delta_e delta_r/1 -> Selector5/1, Selector3/1
  Selector5/1 -> Product1/2
  Selector3/1 -> Product2/2
  Selector6/1 -> Product2/1
  p q r/1 -> Selector9/1, Selector10/1
  Selector9/1 -> Gain1/1
  Selector8/1 -> Product4/2
  Selector7/1 -> Product3/2
  Selector10/1 -> Gain/1
  Gain/1 -> Product3/1
  Gain1/1 -> Product4/1
  Selector11/1 -> Divide/2, Divide1/2
  Product4/1 -> Divide1/1
  Product3/1 -> Divide/1
  Product/1 -> Add/1
  Product1/1 -> Add/2
  Product2/1 -> Add/3
  Divide/1 -> Add/4
  Divide1/1 -> Add/5
  Add/1 -> Product5/2
  QS/1 -> Gain2/1
  Gain2/1 -> Product5/1
  delta_p/1 -> airdata/2(delta_p), Calculate ETA/3, Product6/1
  Product5/1 -> Add1/1
  Add1/1 -> L/1
  Calculate ETA/1 -> Gain3/1
  [Alt] -> Calculate ETA/1
  Selector12/1 -> Calculate ETA/2
  Gain3/1 -> M_aero_D/1
  Thrust/1 -> Gain4/1
  Gain4/1 -> Product6/2
  Product6/1 -> M_aero_D/2
  M_aero_D/1 -> Gain5/1
  Gain5/1 -> Add1/2
  delta_flap/1 -> airdata/3(delta_flap)

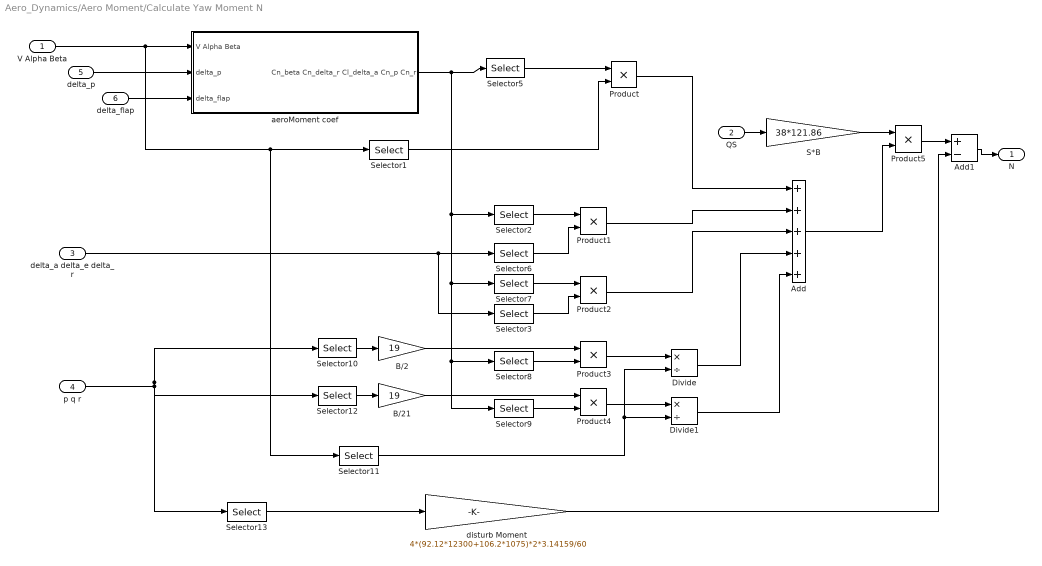
== system Aero_Dynamics/Aero Moment/Calculate Yaw Moment N ==
  V Alpha Beta : Inport
  QS : Inport  Port=2
  delta_a delta_e delta_r : Inport  Port=3
  p q r : Inport  Port=4
  delta_p : Inport  Port=5
  delta_flap : Inport  Port=6
  Add : Sum  Inputs=+++++
  Add1 : Sum  Inputs=+-
  B/2 : Gain  Gain=19
  B/21 : Gain  Gain=19
  Divide : Product  Inputs=*/
  Divide1 : Product  Inputs=*/
  Product{,1..5} (6 alike) : Product  RndMeth=Zero
  S*B : Gain  Gain=38*121.86
  Selector1 : Selector  InputPortWidth=3  Indices=[3]  OutputSizes=[(-2)]
  Selector10 : Selector  InputPortWidth=3  Indices=[1]  OutputSizes=[(-2)]
  Selector11 : Selector  InputPortWidth=3  Indices=[1]  OutputSizes=[(-2)]
  Selector12 : Selector  InputPortWidth=3  Indices=[3]  OutputSizes=[(-2)]
  Selector13 : Selector  InputPortWidth=3  Indices=[2]  OutputSizes=[(-2)]
  Selector2 : Selector  InputPortWidth=5  Indices=[2]  OutputSizes=[(-2)]
  Selector3 : Selector  InputPortWidth=3  Indices=[1]  OutputSizes=[(-2)]
  Selector5 : Selector  InputPortWidth=5  Indices=[1]  OutputSizes=[(-2)]
  Selector6 : Selector  InputPortWidth=3  Indices=[3]  OutputSizes=[(-2)]
  Selector7 : Selector  InputPortWidth=5  Indices=[3]  OutputSizes=[(-2)]
  Selector8 : Selector  InputPortWidth=5  Indices=[4]  OutputSizes=[(-2)]
  Selector9 : Selector  InputPortWidth=5  Indices=[5]  OutputSizes=[(-2)]
  aeroMoment coef : Subsystem
  disturb Moment : Gain  Gain=4*(92.12*12300+106.2*1075)*2*3.14159/60
  N : Outport
  wires:
  V Alpha Beta/1 -> aeroMoment coef/1(V Alpha Beta), Selector1/1, Selector11/1
  delta_p/1 -> aeroMoment coef/2(delta_p)
  aeroMoment coef/1(Cn_beta Cn_delta_r Cl_delta_a Cn_p Cn_r) -> Selector5/1, Selector2/1, Selector7/1, Selector8/1, Selector9/1
  Selector5/1 -> Product/1
  Selector1/1 -> Product/2
  Selector2/1 -> Product1/1
  delta_a delta_e delta_r/1 -> Selector6/1, Selector3/1
  Selector6/1 -> Product1/2
  Selector3/1 -> Product2/2
  Selector7/1 -> Product2/1
  p q r/1 -> Selector12/1, Selector10/1, Selector13/1
  Selector12/1 -> B/21/1
  Selector9/1 -> Product4/2
  Selector8/1 -> Product3/2
  Selector10/1 -> B/2/1
  B/2/1 -> Product3/1
  B/21/1 -> Product4/1
  Selector11/1 -> Divide/2, Divide1/2
  Product4/1 -> Divide1/1
  Product3/1 -> Divide/1
  Product/1 -> Add/1
  Product1/1 -> Add/2
  Product2/1 -> Add/3
  Divide/1 -> Add/4
  Divide1/1 -> Add/5
  Add/1 -> Product5/2
  QS/1 -> S*B/1
  S*B/1 -> Product5/1
  Product5/1 -> Add1/1
  Add1/1 -> N/1
  Selector13/1 -> disturb Moment/1
  disturb Moment/1 -> Add1/2
  delta_flap/1 -> aeroMoment coef/3(delta_flap)

== system Aero_Dynamics/Aero Moment/Calculate pitch Moment M ==
  QS : Inport
  V alpha beta : Inport  Port=2
  delta_p : Inport  Port=3
  delta_a delta_e delta_r : Inport  Port=4
  p q r : Inport  Port=5
  Thrust : Inport  Port=6
  delta_flap : Inport  Port=7
  CA2 : Gain  Gain=CA*121.86
  CA4 : Gain  Gain=-2*(0.5208+0.5909)*9.8
  "Caculate CM " : Subsystem
  Calculate Delta_M : Subsystem
  Product4 : Product  RndMeth=Zero
  Selector13 : Selector  InputPortWidth=3  Indices=[3]  OutputSizes=[(-2)]
  Selector2 : Selector  InputPortWidth=3  Indices=[1 2 ]  OutputSizes=[(-2)]
  Selector3 : Selector  InputPortWidth=3  Indices=[2]  OutputSizes=[(-2)]
  Selector9 : Selector  InputPortWidth=3  Indices=[2]  OutputSizes=[(-2)]
  Sum4 : Sum  Inputs=++++
  disturb Moment : Gain  Gain=4*(92.12*12300+106.2*1075)*2*3.14159/60
  M : Outport
  wires:
  V alpha beta/1 -> Selector2/1
  delta_a delta_e delta_r/1 -> Selector3/1
  delta_p/1 -> "Caculate CM "/2(delta_p)
  p q r/1 -> Selector9/1, Selector13/1
  Selector9/1 -> "Caculate CM "/4(q)
  QS/1 -> CA2/1, Calculate Delta_M/2(Qs)
  CA2/1 -> Product4/1
  Product4/1 -> Sum4/1
  Thrust/1 -> CA4/1, Calculate Delta_M/3(Thrust)
  CA4/1 -> Sum4/2
  Selector13/1 -> disturb Moment/1
  disturb Moment/1 -> Sum4/4
  Sum4/1 -> M/1
  "Caculate CM "/1(Cm) -> Product4/2
  Selector3/1 -> "Caculate CM "/3(delta_e)
  Selector2/1 -> "Caculate CM "/1(" V Alpha"), Calculate Delta_M/1(" V Alpha")
  Calculate Delta_M/1(DelatM) -> Sum4/3
  delta_flap/1 -> "Caculate CM "/5(delta_flap)

== system Aero_Dynamics/RusPlane/AV Alpha Beta ==
  udot vdot wdot : Inport
  Alpha dot : Fcn  Expr="(  - u[1]*u[6] + u[3]*u[4]  ) / ( u[4]*u[4]+ u[6]*u[6] )"
  Beta dot : Fcn  Expr="( u[7]*u[2]-u[5]*( (  u[1]*u[4] + u[2]*u[5] + u[3]*u[6] ) / u[7] ) ) / ( cos(u[9])*u[7]*u[7] )"
  Mux : Mux  Inputs=3
  Mux1 : Mux  Inputs=[3 3 3]
  Mux2 : Mux  Inputs=3
  V  alpha beta : Integrator  InitialCondition=Vab_0
  V dot : Fcn  Expr="(  u[1]*u[4] + u[2]*u[5] + u[3]*u[6] ) / u[7]"
  "Vx " : Fcn  Expr=u[1]*cos(u[2])*cos(u[3])
  Vy1 : Fcn  Expr=u[1]*sin(u[2])*cos(u[3])
  Vz1 : Fcn  Expr=u[1]*sin(u[3])
  V alpha beta : Outport  InitialOutput=0
  u v w  in : Outport  Port=2  InitialOutput=0
  wires:
  Mux2/1 -> V  alpha beta/1
  V dot/1 -> Mux2/1
  Alpha dot/1 -> Mux2/2
  Beta dot/1 -> Mux2/3
  udot vdot wdot/1 -> Mux1/1
  Mux1/1 -> Alpha dot/1, V dot/1, Beta dot/1
  V  alpha beta/1 -> V alpha beta/1, Mux1/3, "Vx "/1, Vz1/1, Vy1/1
  Mux/1 -> Mux1/2, u v w  in/1
  "Vx "/1 -> Mux/1  "u"
  Vz1/1 -> Mux/2  "v"
  Vy1/1 -> Mux/3  "w"

== system Aero_Dynamics/RusPlane/Calculate DCM & Euler Angles ==
  "Wxyz " : Inport
  phi theta psi : Integrator  InitialCondition=eul_0
  phidot psidot thetadot : Subsystem
  Euler : Outport
  wires:
  "Wxyz "/1 -> phidot psidot thetadot/1(Wx Wy Wz)
  phidot psidot thetadot/1(phidot thetadot psidot) -> phi theta psi/1
  phi theta psi/1 -> Euler/1, phidot psidot thetadot/2(phi theta psi)

== system Aero_Dynamics/RusPlane/Subsystem ==
  Moment L M N : Inport
  pqr : Inport  Port=2
  inertia Ix Iy Iz Ixz : Inport  Port=3
  Beta dot : Fcn  Expr="( u[7]*u[3]+  u[1]*u[10] +  u[5]*u[6]*u[10]*(  u[8]-u[9]-u[7] )+  u[4]*u[5]*(  u[7]^2 - u[10]^2-u[7]*u[8]) ) / (u[7]*u[9]-u[10]^2)"
  Mux1 : Mux  Inputs=[3 3 4]
  Mux2 : Mux  Inputs=3
  p dot : Fcn  Expr=(u[1]*u[9] + u[3]*u[10] +u[4]*u[5]*u[10]* (u[7]+u[9]-u[8])-u[5]*u[6]*(u[9]^2+u[10]^2-u[8]*u[9])) / (u[7]*u[9]-u[10]^2)
  q dot : Fcn  Expr="( u[2]-u[4]*u[6]*(u[7]-u[9]) - u[10]*(u[4]^2-u[6]^2)  ) / u[8]"
  pdot qdot rdot : Outport
  wires:
  Mux1/1 -> Beta dot/1, p dot/1, q dot/1
  Mux2/1 -> pdot qdot rdot/1
  Beta dot/1 -> Mux2/3
  q dot/1 -> Mux2/2
  p dot/1 -> Mux2/1
  inertia Ix Iy Iz Ixz/1 -> Mux1/3
  pqr/1 -> Mux1/2
  Moment L M N/1 -> Mux1/1

== system Aero_Dynamics/RusPlane/Subsystem1 ==
  "U V W " : Inport
  Euler phi  theta  psi : Inport  Port=2
  Mux1 : Mux  Inputs=[3 3 ]
  Mux2 : Mux  Inputs=3
  Xe dot : Fcn  Expr="u[1]*cos(u[5])*cos(u[6])  +   u[2]*(sin(u[4])*sin(u[5]) *cos(u[6])-cos(u[4])*sin(u[6]) )  +u[3]*(sin(u[4])*sin(u[6])+cos(u[4])*sin(u[5])*cos(u[6])  )"
  Ye dot : Fcn  Expr="u[1]*cos(u[5])*sin(u[6])  + u[2]*(sin(u[4])*sin(u[5])*sin(u[6]) + cos(u[4])*cos(u[6]) )  + u[3]*( cos(u[4])*sin(u[5])*sin(u[6])-sin(u[4])*cos(u[6]) )"
  Ze dot : Fcn  Expr="u[2]*sin(u[4])*cos(u[5])  + u[3]*cos(u[4])*cos(u[5]) -u[1]*sin(u[5])"
  Xedot Yedot Zedot : Outport
  wires:
  Xe dot/1 -> Mux2/1
  Ze dot/1 -> Mux2/3
  Mux2/1 -> Xedot Yedot Zedot/1
  "U V W "/1 -> Mux1/1
  Euler phi  theta  psi/1 -> Mux1/2
  Mux1/1 -> Xe dot/1, Ye dot/1, Ze dot/1
  Ye dot/1 -> Mux2/2

== system Aero_Dynamics/Aero Force/Caculate Y/Cy_beta ==
  Ma : Inport
  alpha : Inport  Port=2
  delta_flap : Inport  Port=3
  Add1 : Sum
  Cy_beta0 : Lookup2D  RowIndex=[0 6/57.3]  ColumnIndex=Mach_table  Table=Cybeta0
  Cy_beta_alpha : Lookup2D  RowIndex=[0 6/57.3]  ColumnIndex=Mach_table  Table=Cybtaf
  Product5 : Product  RndMeth=Zero
  Cybeta : Outport
  wires:
  Cy_beta0/1 -> Add1/1
  Cy_beta_alpha/1 -> Product5/1
  Product5/1 -> Add1/2
  Ma/1 -> Cy_beta0/2, Cy_beta_alpha/2
  Add1/1 -> Cybeta/1
  alpha/1 -> Product5/2
  delta_flap/1 -> Cy_beta0/1, Cy_beta_alpha/1

== system Aero_Dynamics/Aero Force/Calculate  Lift/Caculate CL ==
  Alpha : Inport
  delta_e : Inport  Port=2
  delta_flap : Inport  Port=3
  Alpha_0 : Lookup2D  RowIndex=[0 6/57.3]  ColumnIndex=Mach_table  Table=Alpha0
  Cl_alpha : Lookup2D  RowIndex=[0 6/57.3]  ColumnIndex=Mach_table  Table=CLAlpha
  Cl_alpha*alpha : Product  RndMeth=Zero
  Cl_delta_e*delta_e : Product  RndMeth=Zero
  Cldelta_e : Lookup2D  RowIndex=[0 6/57.3]  ColumnIndex=Mach_table  Table=CLDelE
  Constant : Constant  Value=4/57.3
  Subtract : Sum
  Subtract1 : Sum  Inputs=+-
  Subtract2 : Sum
  CL : Outport
  wires:
  Cldelta_e/1 -> Cl_delta_e*delta_e/1
  delta_e/1 -> Cl_delta_e*delta_e/2
  Constant/1 -> Subtract/1
  Alpha/1 -> Subtract/2
  [Ma] -> Alpha_0/2, Cldelta_e/2, Cl_alpha/2
  Subtract/1 -> Subtract1/1
  Alpha_0/1 -> Subtract1/2
  Cl_alpha/1 -> Cl_alpha*alpha/1
  Subtract1/1 -> Cl_alpha*alpha/2
  Cl_alpha*alpha/1 -> Subtract2/1
  Cl_delta_e*delta_e/1 -> Subtract2/2
  Subtract2/1 -> CL/1
  delta_flap/1 -> Cl_alpha/1, Alpha_0/1, Cldelta_e/1

== system Aero_Dynamics/Aero Force/Calculate  Lift/SlipStream Strength B ==
  Thrust : Inport
  Qs : Inport  Port=2
  Divide : Product  Inputs=*/
  S : Gain  Gain=12.566
  B : Outport
  wires:
  S/1 -> Divide/2
  Qs/1 -> S/1
  Divide/1 -> B/1
  Thrust/1 -> Divide/1

== system Aero_Dynamics/Aero Force/Calculate  Lift/alpha_w_deg ==
  In1 : Inport
  Constant : Constant  Value=4
  S3 : Gain  Gain=57.3
  Subtract : Sum
  Out1 : Outport
  wires:
  S3/1 -> Subtract/1
  Constant/1 -> Subtract/2
  In1/1 -> S3/1
  Subtract/1 -> Out1/1

== system Aero_Dynamics/Aero Force/Calculate Drag/Caculate CD  ==
  " delta_flap" : Inport
  "  Alpha_w" : Inport  Port=2
  AD : Lookup2D  RowIndex=[0 6/57.3]  ColumnIndex=Mach_table  Table=AD
  Add : Sum
  Alpha0 : Lookup2D  RowIndex=[0 6/57.3]  ColumnIndex=Mach_table  Table=Alpha0
  CDmin : Lookup2D  RowIndex=[0 6/57.3]  ColumnIndex=Mach_table  Table=CDmin
  CLDM : Lookup2D  RowIndex=[0 6/57.3]  ColumnIndex=Mach_table  Table=CLDM
  Cl_alpha : Lookup2D  RowIndex=[0 6/57.3]  ColumnIndex=Mach_table  Table=CLAlpha
  Product : Product  RndMeth=Zero
  Product1 : Product  RndMeth=Zero
  Product2 : Product  RndMeth=Zero
  Subtract : Sum  Inputs=+-
  alpha_w-alpha0 : Sum  Inputs=-+
  CD : Outport
  wires:
  [Ma] -> Alpha0/2, CLDM/2, Cl_alpha/2, AD/2, CDmin/2
  CDmin/1 -> Add/1
  "  Alpha_w"/1 -> alpha_w-alpha0/2
  Alpha0/1 -> alpha_w-alpha0/1
  alpha_w-alpha0/1 -> Product/2
  Cl_alpha/1 -> Product/1
  Product/1 -> Subtract/1
  CLDM/1 -> Subtract/2
  Subtract/1 -> Product1/1, Product1/2
  AD/1 -> Product2/1
  Product1/1 -> Product2/2
  Product2/1 -> Add/2
  Add/1 -> CD/1
  " delta_flap"/1 -> CDmin/1, AD/1, Cl_alpha/1, Alpha0/1, CLDM/1

== system Aero_Dynamics/Aero Force/Calculate Drag/SlipStream Strength B ==
  Thrust : Inport
  Qs : Inport  Port=2
  Divide : Product  Inputs=*/
  S : Gain  Gain=12.566
  B : Outport
  wires:
  S/1 -> Divide/2
  Qs/1 -> S/1
  Divide/1 -> B/1
  Thrust/1 -> Divide/1

== system Aero_Dynamics/Aero Force/Calculate Drag/alpha_w_deg ==
  In1 : Inport
  Constant : Constant  Value=4
  S3 : Gain  Gain=57.3
  Subtract : Sum
  Out1 : Outport
  wires:
  S3/1 -> Subtract/1
  Constant/1 -> Subtract/2
  In1/1 -> S3/1
  Subtract/1 -> Out1/1

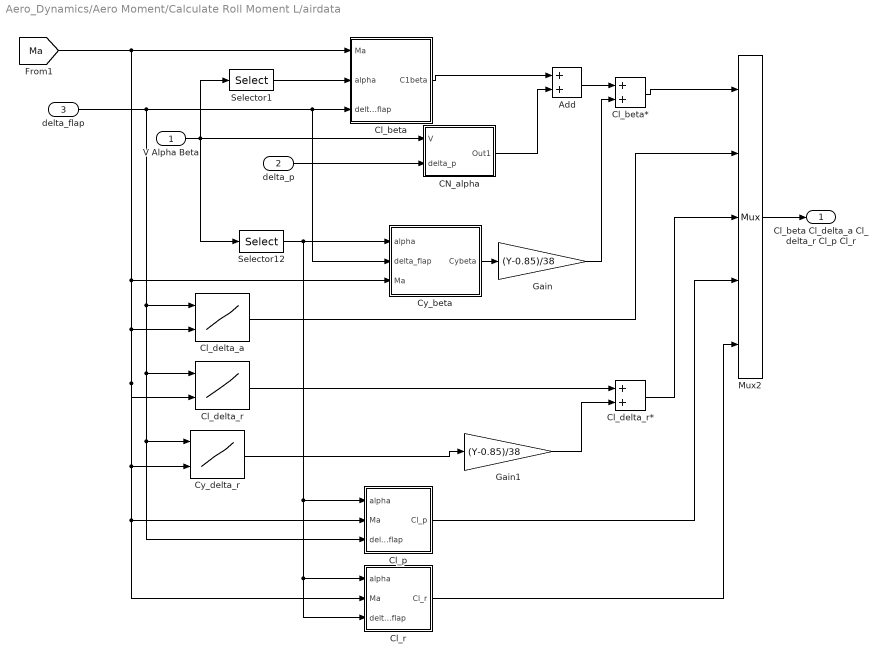
== system Aero_Dynamics/Aero Moment/Calculate Roll Moment L/airdata ==
  V Alpha Beta : Inport
  delta_p : Inport  Port=2
  delta_flap : Inport  Port=3
  Add : Sum
  CN_alpha : Subsystem
  Cl_beta : Subsystem
  Cl_beta* : Sum
  Cl_delta_a : Lookup2D  RowIndex=[0 6/57.3]  ColumnIndex=Mach_table  Table=ClDelA
  Cl_delta_r : Lookup2D  RowIndex=[0 6/57.3]  ColumnIndex=Mach_table  Table=ClDelR
  Cl_delta_r* : Sum
  Cl_p : Subsystem
  Cl_r : Subsystem
  Cy_beta : Subsystem
  Cy_delta_r : Lookup2D  RowIndex=[0 6/57.3]  ColumnIndex=Mach_table  Table=CyDelR
  Gain : Gain  Gain=(Y-0.85)/38
  Gain1 : Gain  Gain=(Y-0.85)/38
  Mux2 : Mux  Inputs=5
  Selector1 : Selector  InputPortWidth=3  Indices=[2]  OutputSizes=[(-2)]
  Selector12 : Selector  InputPortWidth=3  Indices=[2]  OutputSizes=[(-2)]
  Cl_beta Cl_delta_a Cl_delta_r Cl_p Cl_r : Outport
  wires:
  [Ma] -> Cl_p/2(Ma), Cl_r/2(Ma), Cy_delta_r/2, Cl_delta_r/2, Cl_delta_a/2, Cy_beta/3(Ma), Cl_beta/1(Ma)
  Mux2/1 -> Cl_beta Cl_delta_a Cl_delta_r Cl_p Cl_r/1
  delta_p/1 -> CN_alpha/2(delta_p)
  V Alpha Beta/1 -> CN_alpha/1(V), Selector12/1, Selector1/1
  CN_alpha/1(Out1) -> Add/2
  Cy_beta/1(Cybeta) -> Gain/1
  Gain/1 -> Cl_beta*/2
  Add/1 -> Cl_beta*/1
  Cy_delta_r/1 -> Gain1/1
  Cl_delta_r/1 -> Cl_delta_r*/1
  Gain1/1 -> Cl_delta_r*/2
  Cl_beta*/1 -> Mux2/1
  Cl_delta_a/1 -> Mux2/2
  Cl_delta_r*/1 -> Mux2/3
  Cl_p/1(Cl_p) -> Mux2/4
  Cl_r/1(Cl_r) -> Mux2/5
  Selector12/1 -> Cl_p/1(alpha), Cl_r/1(alpha), Cl_r/3(delta_flap), Cy_beta/1(alpha)
  Cl_beta/1(C1beta) -> Add/1
  Selector1/1 -> Cl_beta/2(alpha)
  delta_flap/1 -> Cl_beta/3(delta_flap), Cy_beta/2(delta_flap), Cl_delta_a/1, Cl_delta_r/1, Cy_delta_r/1, Cl_p/3(delta_flap)
